simulink model "gm_mpu6050"  (R2017a)
settings: Solver=FixedStepDiscrete  StartTime=0.0  StopTime=0.004  RelTol=1e-3
PostLoadFcn:
  | ChipSelect = 1;  % choose I2C comms
  | AddressAlt = 0;  % use default address
  | 
  | if AddressAlt == 1
  | % b1101001 (pin AD0 is logic high).
  | SlvAddr = uint8(bin2dec('1101001'));  % ADDR ALT = 1
  | else
  | % b1101000 (pin AD0 is logic low)
  | SlvAddr = uint8(bin2dec('1101000'));  % ADDR ALT = 0
  | end
  | SlvAddr = uint8(hex2dec('68'));
  | 
  | 
  | % 0x3B 59 ACCEL_XOUT[15:8]
  | % 0x3C 60 ACCEL_XOUT[7:0]
  | % 0x3D 61 ACCEL_YOUT[15:8]
  | % 0x3E 62 ACCEL_YOUT[7:0]
  | % 0x3F 63 ACCEL_ZOUT[15:8]
  | % 0x40 64 ACCEL_ZOUT[7:0]
  | 
  | AccelXRegAddr = uint8(hex2dec('3B'));
  | AccelYRegAddr = uint8(hex2dec('3D'));
  | AccelZRegAddr = uint8(hex2dec('3F'));
  | 
  | % 0x43 67 GYRO_XOUT[15:8]
  | % 0x44 68 GYRO_XOUT[7:0]
  | % 0x45 69 GYRO_YOUT[15:8]
  | % 0x46 70 GYRO_YOUT[7:0]
  | % 0x47 71 GYRO_ZOUT[15:8]
  | % 0x48 72 GYRO_ZOUT[7:0]
  | 
  | GyroXRegAddr = uint8(hex2dec('43'));
  | GyroYRegAddr = uint8(hex2dec('45'));
  | GyroZRegAddr = uint8(hex2dec('47'));
  | 
  | deviceAddr = fi(SlvAddr,0,7,0);
  | 
  | powerRegAddr = uint8(hex2dec('6B'));
  | powerRegData = bin2dec('10000001');
settings Model: Creator=skuznick  LastModifiedBy=mini
settings DataIOCC: SaveOutput=off  SaveTime=off
settings OptimizationCC: BlockReduction=off  ConditionallyExecuteInputs=off  DefaultParameterBehavior=Inlined
settings DebuggingCC: AlgebraicLoopMsg=error  InheritedTsInSrcMsg=none  SingleTaskRateTransMsg=error
settings HardwareCC: ProdBitPerPointer=32  ProdBitPerSizeT=32  ProdBitPerPtrDiffT=32  ProdLargestAtomicFloat=None  ProdIntDivRoundTo=Undefined  ProdEndianess=Unspecified  ProdWordSize=32  ProdHWDeviceType=ASIC/FPGA->ASIC/FPGA  ProdEqTarget=off
settings GRTTargetCC: ExtMode=on

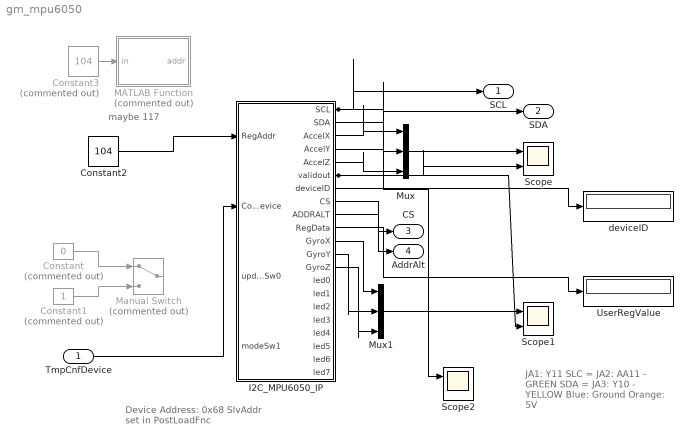
== system gm_mpu6050 ==
  note: Device Address: 0x68
      | SlvAddr set in PostLoadFnc
  note: JA1: Y11
      | SLC = JA2: AA11 - GREEN
      | SDA = JA3: Y10  - YELLOW
      | Blue: Ground
      | Orange: 5V
  note: maybe 117
  TmpCnfDevice : Inport  OutDataTypeStr=boolean
  Constant : Constant  Commented=on  Value=0  OutDataTypeStr=boolean  SampleTime=-1
  Constant1 : Constant  Commented=on  OutDataTypeStr=boolean  SampleTime=-1
  Constant2 : Constant  Value=104  OutDataTypeStr=uint8  SampleTime=-1
  Constant3 : Constant  Commented=on  Value=104  OutDataTypeStr=uint8  SampleTime=-1
  I2C_MPU6050_IP : Subsystem  TreatAsAtomicUnit=on  SystemSampleTime=1/400e3
  MATLAB Function : MATLAB Function  Commented=on  TreatAsAtomicUnit=on
  Manual Switch : ManualSwitch  Commented=on
  Mux : Mux  Inputs=3
  Mux1 : Mux  Inputs=3
  Scope : Scope  NumInputPorts=2
  Scope1 : Scope  NumInputPorts=2
  Scope2 : Scope  NumInputPorts=2
  UserRegValue : Display
  deviceID : Display
  SCL : Outport
  SDA : Outport  Port=2
  CS : Outport  Port=3
  AddrAlt : Outport  Port=4
  wires:
  Constant3/1 -> MATLAB Function/1(in)
  TmpCnfDevice/1 -> I2C_MPU6050_IP/2(ConfigDevice)
  I2C_MPU6050_IP/6(validout) -> Scope1/2, Scope/2
  I2C_MPU6050_IP/12(GyroY) -> Mux1/2
  I2C_MPU6050_IP/11(GyroX) -> Mux1/1
  I2C_MPU6050_IP/13(GyroZ) -> Mux1/3
  Mux1/1 -> Scope1/1
  Constant2/1 -> I2C_MPU6050_IP/1(RegAddr)
  Constant1/1 -> Manual Switch/2
  Constant/1 -> Manual Switch/1
  Mux/1 -> Scope/1
  I2C_MPU6050_IP/10(RegData) -> UserRegValue/1
  I2C_MPU6050_IP/7(deviceID) -> deviceID/1
  I2C_MPU6050_IP/5(AccelZ) -> Mux/3
  I2C_MPU6050_IP/3(AccelX) -> Mux/1
  I2C_MPU6050_IP/4(AccelY) -> Mux/2
  I2C_MPU6050_IP/9(ADDRALT) -> AddrAlt/1
  I2C_MPU6050_IP/8(CS) -> CS/1
  I2C_MPU6050_IP/1(SCL) -> SCL/1, Scope2/1
  I2C_MPU6050_IP/2(SDA) -> SDA/1

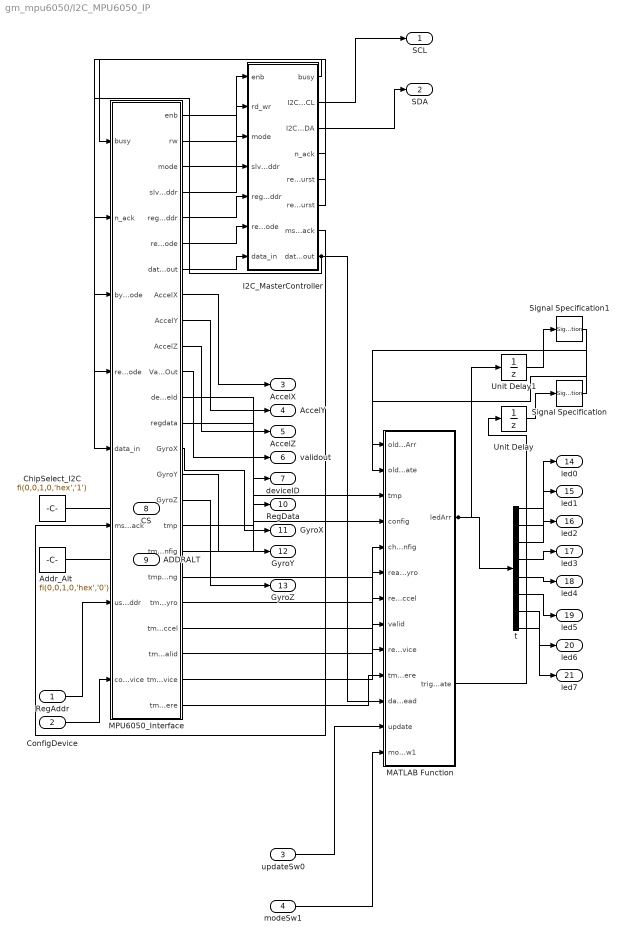
== system gm_mpu6050/I2C_MPU6050_IP ==
  RegAddr : Inport  OutDataTypeStr=uint8  SampleTime=2.5e-06
  ConfigDevice : Inport  Port=2  OutDataTypeStr=boolean  SampleTime=2.5e-06
  updateSw0 : Inport  Port=3  OutDataTypeStr=boolean  SampleTime=2.5e-06
  modeSw1 : Inport  Port=4  OutDataTypeStr=boolean  SampleTime=2.5e-06
  Addr_Alt : Constant  Value=fi(0,0,1,0,'hex','0')  OutDataTypeStr=boolean  SampleTime=-1
  ChipSelect_I2C : Constant  Value=fi(0,0,1,0,'hex','1')  OutDataTypeStr=boolean  SampleTime=-1
  I2C_MasterController : Subsystem
  MATLAB Function : Subsystem
  MPU6050_Interface : Subsystem
  Signal Specification : SignalSpecification  OutDataTypeStr=boolean  Dimensions=1
  Signal Specification1 : SignalSpecification  OutDataTypeStr=boolean  Dimensions=8
  Unit Delay : UnitDelay  SampleTime=2.5e-06
  Unit Delay1 : UnitDelay  SampleTime=2.5e-06
  t : Demux  Outputs=8
  SCL : Outport
  SDA : Outport  Port=2
  AccelX : Outport  Port=3
  AccelY : Outport  Port=4
  AccelZ : Outport  Port=5
  validout : Outport  Port=6
  deviceID : Outport  Port=7
  CS : Outport  Port=8
  ADDRALT : Outport  Port=9
  RegData : Outport  Port=10
  GyroX : Outport  Port=11
  GyroY : Outport  Port=12
  GyroZ : Outport  Port=13
  led0 : Outport  Port=14  OutDataTypeStr=boolean
  led1 : Outport  Port=15  OutDataTypeStr=boolean
  led2 : Outport  Port=16  OutDataTypeStr=boolean
  led3 : Outport  Port=17  OutDataTypeStr=boolean
  led4 : Outport  Port=18  OutDataTypeStr=boolean
  led5 : Outport  Port=19  OutDataTypeStr=boolean
  led6 : Outport  Port=20  OutDataTypeStr=boolean
  led7 : Outport  Port=21  OutDataTypeStr=boolean
  wires:
  RegAddr/1 -> MPU6050_Interface/7(userRegAddr)
  ConfigDevice/1 -> MPU6050_Interface/8(configDevice)
  updateSw0/1 -> MATLAB Function/12(update)
  modeSw1/1 -> MATLAB Function/13(modeSw1)
  Addr_Alt/1 -> ADDRALT/1
  ChipSelect_I2C/1 -> CS/1
  I2C_MasterController/1(busy) -> MPU6050_Interface/1(busy)
  I2C_MasterController/2(I2C_SCL) -> SCL/1
  I2C_MasterController/3(I2C_SDA) -> SDA/1
  I2C_MasterController/4(n_ack) -> MPU6050_Interface/2(n_ack)
  I2C_MasterController/5(reg_data_burst) -> MPU6050_Interface/3(byte_mode)
  I2C_MasterController/6(reg_addr_burst) -> MPU6050_Interface/4(reg_mode)
  I2C_MasterController/7(mstr_ack) -> MPU6050_Interface/6(mstr_ack)
  I2C_MasterController/8(data_out) -> MPU6050_Interface/5(data_in), MATLAB Function/11(dataRead)
  MATLAB Function/1(ledArr) -> t/1, Unit Delay1/1
  MATLAB Function/2(trigUpdate) -> Unit Delay/1
  MPU6050_Interface/1(enb) -> I2C_MasterController/1(enb)
  MPU6050_Interface/2(rw) -> I2C_MasterController/2(rd_wr)
  MPU6050_Interface/3(mode) -> I2C_MasterController/3(mode)
  MPU6050_Interface/4(slv_addr) -> I2C_MasterController/4(slv_addr)
  MPU6050_Interface/5(reg_addr) -> I2C_MasterController/5(reg_addr)
  MPU6050_Interface/6(reg_byte_mode) -> I2C_MasterController/6(reg_byte_mode)
  MPU6050_Interface/7(data_out) -> I2C_MasterController/7(data_in)
  MPU6050_Interface/8(AccelX) -> AccelX/1
  MPU6050_Interface/9(AccelY) -> AccelY/1
  MPU6050_Interface/10(AccelZ) -> AccelZ/1
  MPU6050_Interface/11(Valid_Out) -> validout/1
  MPU6050_Interface/12(deviceId) -> deviceID/1
  MPU6050_Interface/13(regdata) -> RegData/1
  MPU6050_Interface/14(GyroX) -> GyroX/1
  MPU6050_Interface/15(GyroY) -> GyroY/1
  MPU6050_Interface/16(GyroZ) -> GyroZ/1
  MPU6050_Interface/17(tmp) -> MATLAB Function/3(tmp)
  MPU6050_Interface/18(tmpConfig) -> MATLAB Function/4(config)
  MPU6050_Interface/19(tmpCheckCng) -> MATLAB Function/5(checkConfig)
  MPU6050_Interface/20(tmpReadGyro) -> MATLAB Function/6(readGyro)
  MPU6050_Interface/21(tmpReadAccel) -> MATLAB Function/7(readAccel)
  MPU6050_Interface/22(tmpValid) -> MATLAB Function/8(valid)
  MPU6050_Interface/23(tmpReadDevice) -> MATLAB Function/9(readDevice)
  MPU6050_Interface/24(tmpHere) -> MATLAB Function/10(tmpHere)
  Signal Specification/1 -> MATLAB Function/2(oldTrigUpdate)
  Signal Specification1/1 -> MATLAB Function/1(oldLedArr)
  Unit Delay/1 -> Signal Specification/1
  Unit Delay1/1 -> Signal Specification1/1
  t/1 -> led0/1
  t/2 -> led1/1
  t/3 -> led2/1
  t/4 -> led3/1
  t/5 -> led4/1
  t/6 -> led5/1
  t/7 -> led6/1
  t/8 -> led7/1

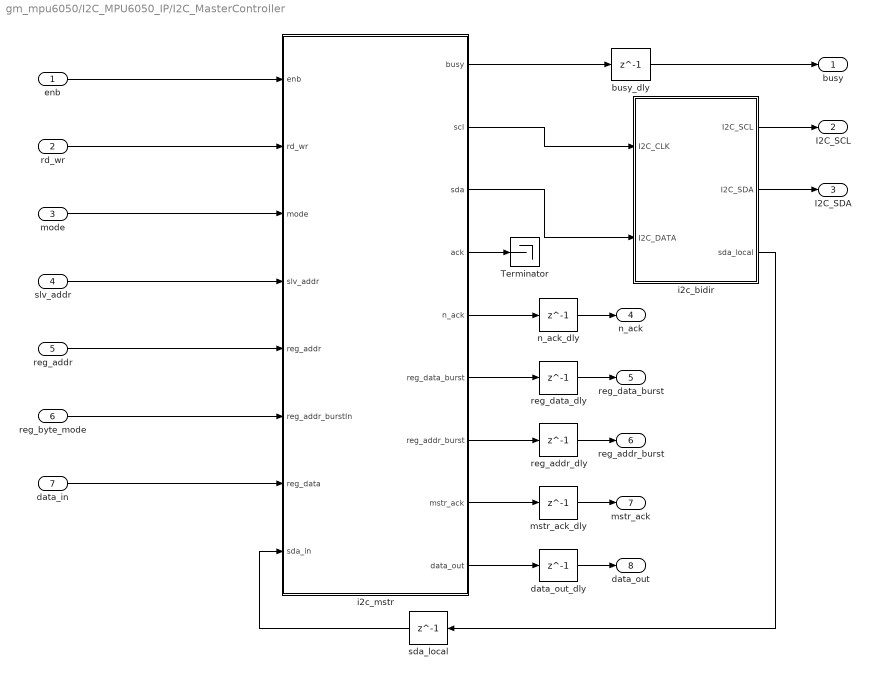
== system gm_mpu6050/I2C_MPU6050_IP/I2C_MasterController ==
  enb : Inport  SampleTime=2.5e-06
  rd_wr : Inport  Port=2  SampleTime=2.5e-06
  mode : Inport  Port=3  SampleTime=2.5e-06
  slv_addr : Inport  Port=4  SampleTime=2.5e-06
  reg_addr : Inport  Port=5  SampleTime=2.5e-06
  reg_byte_mode : Inport  Port=6  SampleTime=2.5e-06
  data_in : Inport  Port=7  SampleTime=2.5e-06
  Terminator : Terminator
  busy_dly : Delay  DelayLength=1
  data_out_dly : Delay  DelayLength=1
  i2c_bidir : Subsystem  TreatAsAtomicUnit=on
  i2c_mstr : Subsystem
  mstr_ack_dly : Delay  DelayLength=1
  n_ack_dly : Delay  DelayLength=1
  reg_addr_dly : Delay  DelayLength=1
  reg_data_dly : Delay  DelayLength=1
  sda_local : Delay  DelayLength=1
  busy : Outport
  I2C_SCL : Outport  Port=2
  I2C_SDA : Outport  Port=3
  n_ack : Outport  Port=4
  reg_data_burst : Outport  Port=5
  reg_addr_burst : Outport  Port=6
  mstr_ack : Outport  Port=7
  data_out : Outport  Port=8
  wires:
  enb/1 -> i2c_mstr/1(enb)
  rd_wr/1 -> i2c_mstr/2(rd_wr)
  mode/1 -> i2c_mstr/3(mode)
  slv_addr/1 -> i2c_mstr/4(slv_addr)
  reg_addr/1 -> i2c_mstr/5(reg_addr)
  reg_byte_mode/1 -> i2c_mstr/6(reg_addr_burstIn)
  data_in/1 -> i2c_mstr/7(reg_data)
  busy_dly/1 -> busy/1
  data_out_dly/1 -> data_out/1
  i2c_bidir/1(I2C_SCL) -> I2C_SCL/1
  i2c_bidir/2(I2C_SDA) -> I2C_SDA/1
  i2c_bidir/3(sda_local) -> sda_local/1
  i2c_mstr/1(busy) -> busy_dly/1
  i2c_mstr/2(scl) -> i2c_bidir/1(I2C_CLK)
  i2c_mstr/3(sda) -> i2c_bidir/2(I2C_DATA)
  i2c_mstr/4(ack) -> Terminator/1
  i2c_mstr/5(n_ack) -> n_ack_dly/1
  i2c_mstr/6(reg_data_burst) -> reg_data_dly/1
  i2c_mstr/7(reg_addr_burst) -> reg_addr_dly/1
  i2c_mstr/8(mstr_ack) -> mstr_ack_dly/1
  i2c_mstr/9(data_out) -> data_out_dly/1
  mstr_ack_dly/1 -> mstr_ack/1
  n_ack_dly/1 -> n_ack/1
  reg_addr_dly/1 -> reg_addr_burst/1
  reg_data_dly/1 -> reg_data_burst/1
  sda_local/1 -> i2c_mstr/8(sda_in)

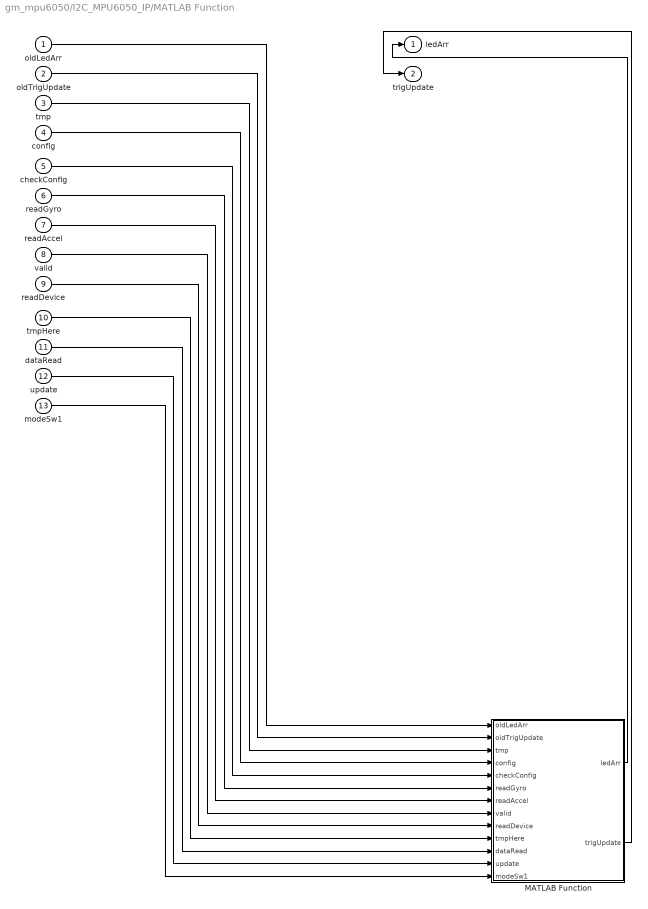
== system gm_mpu6050/I2C_MPU6050_IP/MATLAB Function ==
  oldLedArr : Inport  PortDimensions=[1, 8]  SampleTime=2.5e-06
  oldTrigUpdate : Inport  Port=2  SampleTime=2.5e-06
  tmp : Inport  Port=3  SampleTime=2.5e-06
  config : Inport  Port=4  SampleTime=2.5e-06
  checkConfig : Inport  Port=5  SampleTime=2.5e-06
  readGyro : Inport  Port=6  SampleTime=2.5e-06
  readAccel : Inport  Port=7  SampleTime=2.5e-06
  valid : Inport  Port=8  SampleTime=2.5e-06
  readDevice : Inport  Port=9  SampleTime=2.5e-06
  tmpHere : Inport  Port=10  SampleTime=2.5e-06
  dataRead : Inport  Port=11  SampleTime=2.5e-06
  update : Inport  Port=12  SampleTime=2.5e-06
  modeSw1 : Inport  Port=13  SampleTime=2.5e-06
  MATLAB Function : MATLAB Function  TreatAsAtomicUnit=on
  ledArr : Outport
  trigUpdate : Outport  Port=2
  wires:
  oldLedArr/1 -> MATLAB Function/1(oldLedArr)
  oldTrigUpdate/1 -> MATLAB Function/2(oldTrigUpdate)
  tmp/1 -> MATLAB Function/3(tmp)
  config/1 -> MATLAB Function/4(config)
  checkConfig/1 -> MATLAB Function/5(checkConfig)
  readGyro/1 -> MATLAB Function/6(readGyro)
  readAccel/1 -> MATLAB Function/7(readAccel)
  valid/1 -> MATLAB Function/8(valid)
  readDevice/1 -> MATLAB Function/9(readDevice)
  tmpHere/1 -> MATLAB Function/10(tmpHere)
  dataRead/1 -> MATLAB Function/11(dataRead)
  update/1 -> MATLAB Function/12(update)
  modeSw1/1 -> MATLAB Function/13(modeSw1)
  MATLAB Function/1(ledArr) -> ledArr/1
  MATLAB Function/2(trigUpdate) -> trigUpdate/1

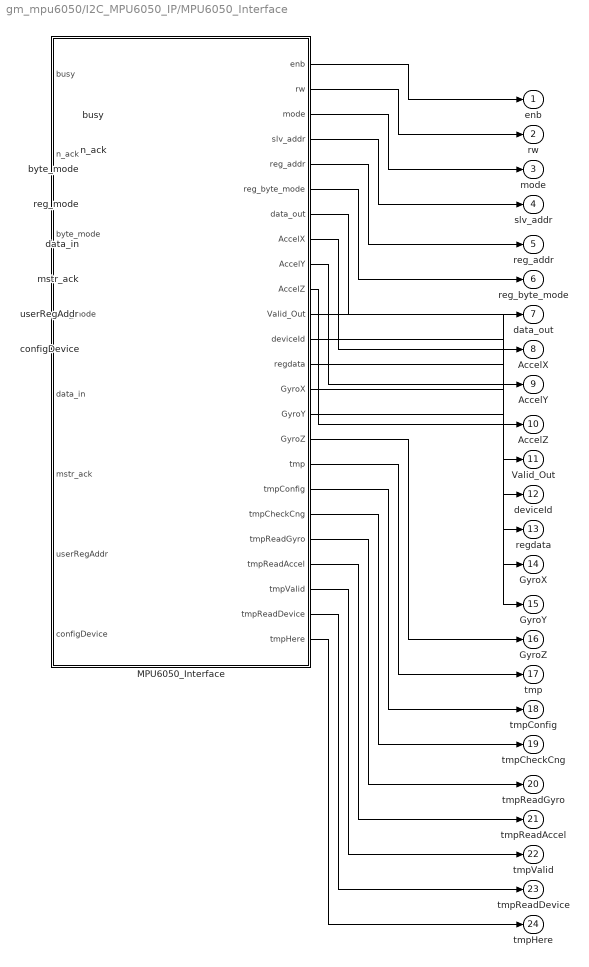
== system gm_mpu6050/I2C_MPU6050_IP/MPU6050_Interface ==
  busy : Inport  SampleTime=2.5e-06
  n_ack : Inport  Port=2  SampleTime=2.5e-06
  byte_mode : Inport  Port=3  SampleTime=2.5e-06
  reg_mode : Inport  Port=4  SampleTime=2.5e-06
  data_in : Inport  Port=5  SampleTime=2.5e-06
  mstr_ack : Inport  Port=6  SampleTime=2.5e-06
  userRegAddr : Inport  Port=7  SampleTime=2.5e-06
  configDevice : Inport  Port=8  SampleTime=2.5e-06
  MPU6050_Interface : Stateflow chart  TreatAsAtomicUnit=on
  enb : Outport
  rw : Outport  Port=2
  mode : Outport  Port=3
  slv_addr : Outport  Port=4
  reg_addr : Outport  Port=5
  reg_byte_mode : Outport  Port=6
  data_out : Outport  Port=7
  AccelX : Outport  Port=8
  AccelY : Outport  Port=9
  AccelZ : Outport  Port=10
  Valid_Out : Outport  Port=11
  deviceId : Outport  Port=12
  regdata : Outport  Port=13
  GyroX : Outport  Port=14
  GyroY : Outport  Port=15
  GyroZ : Outport  Port=16
  tmp : Outport  Port=17
  tmpConfig : Outport  Port=18
  tmpCheckCng : Outport  Port=19
  tmpReadGyro : Outport  Port=20
  tmpReadAccel : Outport  Port=21
  tmpValid : Outport  Port=22
  tmpReadDevice : Outport  Port=23
  tmpHere : Outport  Port=24
  wires:
  busy/1 -> MPU6050_Interface/1(busy)
  n_ack/1 -> MPU6050_Interface/2(n_ack)
  byte_mode/1 -> MPU6050_Interface/3(byte_mode)
  reg_mode/1 -> MPU6050_Interface/4(reg_mode)
  data_in/1 -> MPU6050_Interface/5(data_in)
  mstr_ack/1 -> MPU6050_Interface/6(mstr_ack)
  userRegAddr/1 -> MPU6050_Interface/7(userRegAddr)
  configDevice/1 -> MPU6050_Interface/8(configDevice)
  MPU6050_Interface/1(enb) -> enb/1
  MPU6050_Interface/2(rw) -> rw/1
  MPU6050_Interface/3(mode) -> mode/1
  MPU6050_Interface/4(slv_addr) -> slv_addr/1
  MPU6050_Interface/5(reg_addr) -> reg_addr/1
  MPU6050_Interface/6(reg_byte_mode) -> reg_byte_mode/1
  MPU6050_Interface/7(data_out) -> data_out/1
  MPU6050_Interface/8(AccelX) -> AccelX/1
  MPU6050_Interface/9(AccelY) -> AccelY/1
  MPU6050_Interface/10(AccelZ) -> AccelZ/1
  MPU6050_Interface/11(Valid_Out) -> Valid_Out/1
  MPU6050_Interface/12(deviceId) -> deviceId/1
  MPU6050_Interface/13(regdata) -> regdata/1
  MPU6050_Interface/14(GyroX) -> GyroX/1
  MPU6050_Interface/15(GyroY) -> GyroY/1
  MPU6050_Interface/16(GyroZ) -> GyroZ/1
  MPU6050_Interface/17(tmp) -> tmp/1
  MPU6050_Interface/18(tmpConfig) -> tmpConfig/1
  MPU6050_Interface/19(tmpCheckCng) -> tmpCheckCng/1
  MPU6050_Interface/20(tmpReadGyro) -> tmpReadGyro/1
  MPU6050_Interface/21(tmpReadAccel) -> tmpReadAccel/1
  MPU6050_Interface/22(tmpValid) -> tmpValid/1
  MPU6050_Interface/23(tmpReadDevice) -> tmpReadDevice/1
  MPU6050_Interface/24(tmpHere) -> tmpHere/1

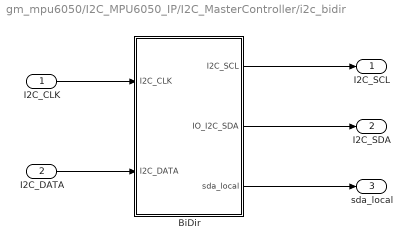
== system gm_mpu6050/I2C_MPU6050_IP/I2C_MasterController/i2c_bidir ==
  I2C_CLK : Inport
  I2C_DATA : Inport  Port=2
  BiDir : Subsystem  TreatAsAtomicUnit=on
  I2C_SCL : Outport
  I2C_SDA : Outport  Port=2
  sda_local : Outport  Port=3
  wires:
  BiDir/3(sda_local) -> sda_local/1
  BiDir/1("I2C_SCL ") -> I2C_SCL/1
  I2C_DATA/1 -> BiDir/2(I2C_DATA)
  I2C_CLK/1 -> BiDir/1(I2C_CLK)
  BiDir/2(IO_I2C_SDA) -> I2C_SDA/1

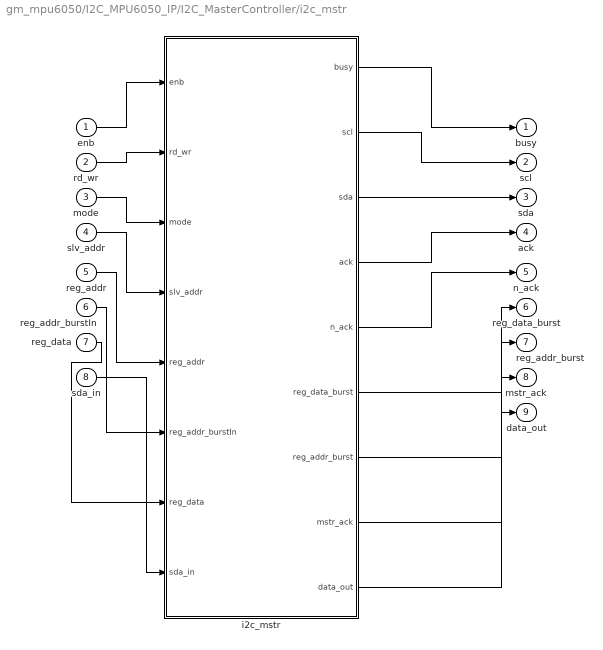
== system gm_mpu6050/I2C_MPU6050_IP/I2C_MasterController/i2c_mstr ==
  enb : Inport  SampleTime=2.5e-06
  rd_wr : Inport  Port=2  SampleTime=2.5e-06
  mode : Inport  Port=3  SampleTime=2.5e-06
  slv_addr : Inport  Port=4  SampleTime=2.5e-06
  reg_addr : Inport  Port=5  SampleTime=2.5e-06
  reg_addr_burstIn : Inport  Port=6  SampleTime=2.5e-06
  reg_data : Inport  Port=7  SampleTime=2.5e-06
  sda_in : Inport  Port=8  SampleTime=2.5e-06
  i2c_mstr : Stateflow chart  TreatAsAtomicUnit=on
  busy : Outport
  scl : Outport  Port=2
  sda : Outport  Port=3
  ack : Outport  Port=4
  n_ack : Outport  Port=5
  reg_data_burst : Outport  Port=6
  reg_addr_burst : Outport  Port=7
  mstr_ack : Outport  Port=8
  data_out : Outport  Port=9
  wires:
  enb/1 -> i2c_mstr/1(enb)
  rd_wr/1 -> i2c_mstr/2(rd_wr)
  mode/1 -> i2c_mstr/3(mode)
  slv_addr/1 -> i2c_mstr/4(slv_addr)
  reg_addr/1 -> i2c_mstr/5(reg_addr)
  reg_addr_burstIn/1 -> i2c_mstr/6(reg_addr_burstIn)
  reg_data/1 -> i2c_mstr/7(reg_data)
  sda_in/1 -> i2c_mstr/8(sda_in)
  i2c_mstr/1(busy) -> busy/1
  i2c_mstr/2(scl) -> scl/1
  i2c_mstr/3(sda) -> sda/1
  i2c_mstr/4(ack) -> ack/1
  i2c_mstr/5(n_ack) -> n_ack/1
  i2c_mstr/6(reg_data_burst) -> reg_data_burst/1
  i2c_mstr/7(reg_addr_burst) -> reg_addr_burst/1
  i2c_mstr/8(mstr_ack) -> mstr_ack/1
  i2c_mstr/9(data_out) -> data_out/1

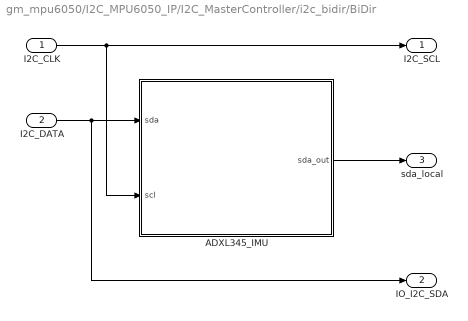
== system gm_mpu6050/I2C_MPU6050_IP/I2C_MasterController/i2c_bidir/BiDir ==
  I2C_CLK : Inport  OutDataTypeStr=boolean
  I2C_DATA : Inport  Port=2  OutDataTypeStr=boolean
  ADXL345_IMU : Stateflow chart  TreatAsAtomicUnit=on
  "I2C_SCL " : Outport  OutDataTypeStr=boolean
  IO_I2C_SDA : Outport  Port=2  OutDataTypeStr=boolean
  sda_local : Outport  Port=3  OutDataTypeStr=boolean
  wires:
  I2C_DATA/1 -> ADXL345_IMU/1(sda), IO_I2C_SDA/1
  I2C_CLK/1 -> ADXL345_IMU/2(scl), "I2C_SCL "/1
  ADXL345_IMU/1(sda_out) -> sda_local/1

== stateflow chart gm_mpu6050/I2C_MPU6050_IP/MPU6050_Interface/MPU6050_Interface ==
  settings: executeAtInitialization=1
  state init
    %initstate
    Valid_Out = 0;
    selfInit = 1;
    slv_addr = SlvAddr;
    %TODO delete all
    tmp = 0;
    tmpConfig = 0;
    tmpReadGyro = 0;
    tmpReadAccel = 0;
    tmpValid = 0;
    tmpReadDevice = 0;
    tmpHere = 0;
  note: I2C Configuration for MPU6050
  note: 0x3B 59 ACCEL_XOUT[15:8]
      | 0x3C 60 ACCEL_XOUT[7:0]
      | 0x3D 61 ACCEL_YOUT[15:8]
      | 0x3E 62 ACCEL_YOUT[7:0]
      | 0x3F 63 ACCEL_ZOUT[15:8]
      | 0x40 64 ACCEL_ZOUT[7:0]
      |
      | 0x43 67 GYRO_XOUT[15:8]
      | 0x44 68 GYRO_XOUT[7:0]
      | 0x45 69 GYRO_YOUT[15:8]
      | 0x46 70 GYRO_YOUT[7:0]
      | 0x47 71 GYRO_ZOUT[15:8]
      | 0x48 72 GYRO_ZOUT[7:0]
      |
      | 0x6B 107 PWR_MGMT_1
      | 0x6C 108 PWR_MGMT_2
  state idle
    %idlestate
    enb 	= 0;
    rw 		= 0;
    mode 	= 0;
    cnt      = 0;
    reg_byte_mode = 0;
  state ReadDeviceData [group]
    note: DEVID is an example of
        | doing a 1-byte READ
    note: 0x75 117 - WHO_AM_I[6:1]
    state getDEVID
      entry:
      enb = 1;
      rw = 1;
      mode = 0;
      reg_addr =   uint8(117);
      tmpReadDevice = 1;
    state waitforNotBusy1
      enb=0;
    state readDEVID
      deviceId = uint8(data_in);
      tmpHere = 1;
    state waitforNotBusy6
      enb=0;
    state getRegData
      entry:
      enb = 1;
      rw = 1;
      mode = 0;
      reg_addr = userRegAddr;
    state waitforNotBusy5
      enb=0;
    state readUserRegData
      regdata = uint8(data_in);
    getDEVID -> waitforNotBusy1 : [busy==1]
    waitforNotBusy1 -> readDEVID [order 1] : [mstr_ack==1]
    waitforNotBusy1 -> waitforNotBusy6 [order 2] : [n_ack==1]
    readDEVID -> getRegData : [busy==0]
    waitforNotBusy6 -> (junction 2281) : [busy==0 || busy == 1]
    getRegData -> waitforNotBusy5 : [busy==1]
    waitforNotBusy5 -> readUserRegData [order 1] : [mstr_ack==1]
    waitforNotBusy5 -> (junction 2281) [order 2] : [n_ack==1]
  state Configuration [group]
    state setPwrMode
      enb = 1;
      rw = 0;
      mode = 0;
      reg_addr = powerRegAddr;
      data_out = powerRegData;
      tmpConfig = 1;
    state waitforNotBusy2
      enb=0;
    state setDataFormat [commented out]
      enb = 1;
      rw = 0;
      mode = 0;
      reg_addr = uint8(49); % 0x31
      data_out = uint8(0); % or 0x08
    state waitforNotBusy3 [commented out]
      enb=0;
    state setFIFOCfg [commented out]
      enb = 1;
      rw = 0;
      mode = 0;
      reg_addr = uint8(56); % 0x38
      data_out = uint8(8); % 0x08
    state waitforNotBusy4 [commented out]
      enb=0;
    state cfgDone
      selfInit = 0;
      tmp = 1;
    setPwrMode -> Configuration.waitforNotBusy2 : [busy==1]
    Configuration.waitforNotBusy2 -> (junction 2329) [order 2] : [busy==0]
    Configuration.waitforNotBusy2 -> (junction 2279) [order 1] : [n_ack==1]
    waitforNotBusy3 -> (junction 2279) [commented out] : [n_ack==1]
    waitforNotBusy4 -> (junction 2279) [commented out] : [n_ack==1]
    setDataFormat -> waitforNotBusy3 [commented out] : [busy==1]
    waitforNotBusy3 -> setFIFOCfg [commented out] : [busy==0]
    (junction 2329) -> cfgDone
    setFIFOCfg -> waitforNotBusy4 [commented out] : [busy==1]
  state check_cfg
    en: enb = 0;
    cnt = 0;
    du: cnt = cnt + 1;
    tmpCheckCng = 1
  state ReadAccelData [group]
    state read_accelX_registers0
      entry:
      enb = 1;
      rw = 1;
      mode = 1;
      reg_addr =  AccelXRegAddr;
      Valid_Out = 0;
      tmpReadAccel = 1;
    state waitforNotBusy2
      enb=0;
    state accelX_LSB
      tempVal = data_in;
    state toggle
    state accelX_MSB
      AccelX =  convert_int16(tempVal, data_in);
    state toggle3
    state accelY_LSB
      tempVal = data_in;
    state toggle1
    state accelY_MSB
      AccelY = convert_int16(tempVal,data_in);
    state toggle4
    state accelZ_LSB
      tempVal = data_in;
    state toggle2
      mode = 0;
    state accelZ_MSB
      AccelZ =  convert_int16(tempVal, data_in);
    read_accelX_registers0 -> ReadAccelData.waitforNotBusy2 : [busy==1]
    ReadAccelData.waitforNotBusy2 -> accelX_LSB [order 1] : [mstr_ack==1]
    accelX_LSB -> ReadAccelData.toggle : [mstr_ack==0]
    ReadAccelData.toggle -> accelX_MSB : [mstr_ack==1]
    accelX_MSB -> ReadAccelData.toggle3 [order 2] : [mstr_ack==0]
    accelX_MSB -> (junction 2286) [order 1] : [n_ack==1]
    ReadAccelData.toggle3 -> accelY_LSB : [mstr_ack==1]
    accelY_LSB -> ReadAccelData.toggle1 : [mstr_ack==0]
    ReadAccelData.toggle1 -> accelY_MSB : [mstr_ack==1]
    accelY_MSB -> (junction 2286) [order 1] : [n_ack==1]
    accelZ_MSB -> (junction 2286) [order 1] : [n_ack==1]
    accelY_MSB -> ReadAccelData.toggle4 [order 2] : [mstr_ack==0]
    ReadAccelData.toggle4 -> accelZ_LSB : [mstr_ack==1]
    accelZ_LSB -> ReadAccelData.toggle2 : [mstr_ack==0]
    ReadAccelData.toggle2 -> accelZ_MSB : [mstr_ack==1]
  state Valid
    en: enb = 0;
    cnt = 0;
    Valid_Out = 1;
    du: cnt = cnt + 1;
    tmpValid = 1;
  state ReadGyroData [group]
    state read_gyroX_registers0
      entry:
      enb = 1;
      rw = 1;
      mode = 1;
      reg_addr =  GyroXRegAddr;
      Valid_Out = 0;
      tmpReadGyro = 1;
    state waitforNotBusy2
      enb=0;
    state gyroX_LSB
      tempVal = data_in;
    state toggle
    state gyroX_MSB
      GyroX =  convert_int16(tempVal, data_in);
    state toggle3
    state gyroY_LSB
      tempVal = data_in;
    state toggle1
    state gyroY_MSB
      GyroY = convert_int16(tempVal, data_in);
    state toggle4
    state gyroZ_LSB
      tempVal = data_in;
    state toggle2
      mode = 0;
    state gyroZ_MSB
      GyroZ =  convert_int16(tempVal, data_in);
    read_gyroX_registers0 -> ReadGyroData.waitforNotBusy2 : [busy==1]
    ReadGyroData.waitforNotBusy2 -> gyroX_LSB : [mstr_ack==1]
    gyroX_LSB -> ReadGyroData.toggle : [mstr_ack==0]
    ReadGyroData.toggle -> gyroX_MSB : [mstr_ack==1]
    gyroX_MSB -> ReadGyroData.toggle3 [order 2] : [mstr_ack==0]
    gyroX_MSB -> (junction 2301) [order 1] : [n_ack==1]
    ReadGyroData.toggle3 -> gyroY_LSB : [mstr_ack==1]
    gyroY_LSB -> ReadGyroData.toggle1 : [mstr_ack==0]
    ReadGyroData.toggle1 -> gyroY_MSB : [mstr_ack==1]
    gyroY_MSB -> (junction 2301) [order 1] : [n_ack==1]
    gyroZ_MSB -> (junction 2301) [order 1] : [n_ack==1]
    gyroY_MSB -> ReadGyroData.toggle4 [order 2] : [mstr_ack==0]
    ReadGyroData.toggle4 -> gyroZ_LSB : [mstr_ack==1]
    gyroZ_LSB -> ReadGyroData.toggle2 : [mstr_ack==0]
    ReadGyroData.toggle2 -> gyroZ_MSB : [mstr_ack==1]
  (default) -> init
  init -> idle
  check_cfg -> idle : [cnt >=5]
  idle -> setPwrMode [order 1] : [busy==0 & (configDevice==1 | selfInit == 1)]
  idle -> getDEVID [order 2] : [busy==0]
  readUserRegData -> read_accelX_registers0 : [busy==0]
  (junction 2281) -> check_cfg
  (junction 2286) -> check_cfg
  (junction 2279) -> check_cfg
  ReadAccelData.waitforNotBusy2 -> check_cfg [order 2] : [n_ack==1]
  Valid -> check_cfg : [cnt >= 5]
  cfgDone -> read_accelX_registers0
  accelZ_MSB -> read_gyroX_registers0 [order 2] : [busy==0]
  gyroZ_MSB -> Valid [order 2]
  data: msb function_input uint8; lsb function_input uint8; val function_output int16; enb output boolean size=1; rw output boolean size=1; mode output boolean size=1; slv_addr output uint8; reg_addr output uint8; reg_byte_mode output boolean size=1; data_out output uint8; busy input; n_ack input; byte_mode input boolean size=1; reg_mode input boolean size=1; cnt local uint32; data_in input uint8 size=1; mstr_ack input; AccelX output int16; AccelY output int16; AccelZ output int16; SlvAddr parameter uint8; AccelXRegAddr parameter uint8; AccelYRegAddr parameter uint8; AccelZRegAddr parameter uint8; Valid_Out output boolean; tempVal local uint8; deviceId output uint8; powerRegData parameter uint8; regdata output uint8; userRegAddr input uint8; powerRegAddr parameter uint8; configDevice input boolean; selfInit local boolean; GyroXRegAddr parameter uint8; GyroX output int16; GyroY output int16; GyroZ output int16; tmp output boolean; tmpConfig output boolean; tmpCheckCng output boolean; tmpReadGyro output boolean; tmpReadAccel output boolean; tmpValid output boolean; tmpReadDevice output boolean; tmpHere output boolean
  function val = convert_int16(msb, lsb):
    | function val = convert_int16(msb, lsb)
    | 
    | val = int16(bitor(bitshift(int16(msb),8), int16(lsb)));

== stateflow chart gm_mpu6050/I2C_MPU6050_IP/I2C_MasterController/i2c_mstr/i2c_mstr ==
  settings: executeAtInitialization=1
  state idle
    entry:
    scl(:) = 1;
    sda(:) = 1;
    busy(:)  = 0;
    reg_data_burst(:) = 0;
    temp_data = uint8(0);
  note: I2C Master Controller
  state stop_ext
    entry:
    scl (:) = 1;
    sda(:) = 1;
    ack(:) = 0;
  state ready
    entry:
    scl(:) = 1;
    sda(:) = 1;
    data_out(:) = 0;
  state stop
    entry:
    sda(:) = 0;
  state start_n
    entry:
    scl(:) = 1;
    sda(:) = 0;
    bit_cnt(:) = 7;
    busy(:) = 1;
    reg_byte_cnt =1;
    data_out(:) = 0;
  state mastr_ack_data_cnf1
    entry:
    scl(:) = 1;
    sda(:) = 1;
    mstr_ack (:) = 1;
  state mastr_ack_data_cnf
    entry:
    scl(:) = 1;
    sda(:) = 0;
    mstr_ack (:) = 1;
  state scl_ext_p
    entry:
    scl(:) = 1;
    sda(:) = 0;
    ack(:) = 0;
  state start_p
    entry:
    sda(:) = 0;
  state scl_ext_n
    entry:
    scl(:) = 0;
    sda(:) = 0;
    ack(:) = 0;
    mstr_ack(:) = 0;
  state mastr_ack_data
    entry:
    scl(:) = 0;
    if mode == 1
    sda(:) = 0; %ACK
    else
    sda(:) = 1; %NACK
    end
    mstr_ack(:) = 1;
    ack(:) = 0;
    data_out(:) = temp_data;
    temp_data(:) = 0;
  state cmd_slave_addr_n
    entry:
    scl(:) = 0;
    sda(:) = bitget(slv_addr(:),bit_cnt);
  state Increment_Byte_count1
    entry:
    scl(:) = 0;
    bit_cnt = 8;
    mstr_ack(:) =0;
    reg_data_burst(:) = 1;
    sda(:) = 1;
  state cmd_slave_addr_p
    entry:
    scl(:) = 1;
    bit_cnt = bit_cnt-1;
  state write_n
    entry:
    scl(:) = 0;
    sda(:) = 0;
  state ack_end1
    entry: scl(:)=1;
    sda(:)=1;
    ack(:)=1;
  state cmd_reg_read_data_p
    entry:
    scl(:) = 1;
    if sda_in == 1;
    temp_data = bitset(temp_data,bit_cnt);
    end
    bit_cnt = bit_cnt-1;
  state ack_end
    entry: scl(:)=1;
    sda(:)=1;
    ack(:)=1;
  state write_p
    entry:
    scl(:) = 1;
    sda(:) = 0;
  state ack_recv_wr3
    entry: scl(:)=1;
    sda(:)=1;
    ack(:)=1;
  state ack_data
    entry:
    scl(:) = 0;
    sda(:) = 1;
    ack(:) = 1;
  state ack_slv
    entry:
    scl(:) = 0;
    ack(:) = 1;
    sda(:) = 1;
  state cmd_reg_read_data_n
    entry:
    scl(:) = 0;
    %mstr_ack(:) = 0
    ack(:) = 1;
  state ack_recv_wr
    entry: scl(:)=1;
    sda(:)=1;
    ack(:)=1;
    bit_cnt = 8;
  state cmd_reg_data_p
    entry:
    scl(:) = 1;
    bit_cnt = bit_cnt-1;
  state ack_addr_m_cnf
    entry:
    scl(:) = 0;
    if rd_wr == 1
    sda(:) = 1;
    else
    sda(:) = 0;
    end
    bit_cnt = 8;
    ack(:) = 0;
  state ack_wr_p
    entry: scl(:)=0;
    ack(:)=0;
    sda(:)=0;
    bit_cnt = 8;
  state error_ack
    entry:
    scl(:) = 0;
    sda(:) = 1;
    n_ack(:) = 1;
  state cmd_reg_data_n
    entry:
    scl(:) = 0;
    ack(:) = 0;
    reg_data_burst(:) = 0;
    sda(:) = bitget(reg_data,bit_cnt);
  state delay
    entry:
    scl(:) = 0;
    sda(:) = 1;
  state cmd_reg_addr_n
    entry:
    scl(:) = 0;
    ack(:) = 0;
    sda(:) = bitget(reg_addr,bit_cnt);
    reg_addr_burst(:)=0;
  state repeat_strt_n
    entry:
    scl(:) = 1;
    sda(:) = 0;
    bit_cnt(:) = 7;
    busy(:) = 1;
    reg_byte_cnt =1;
  state ready_repeated
    entry:
    scl(:) = 1;
    sda(:) = 1;
  state cmd_reg_addr_p
    entry:
    scl(:)= 1;
    bit_cnt = bit_cnt-1;
  state repeat_strt_p
    entry:
    sda(:) = 0;
  state ready_repeated_dummy
    entry:
    scl(:) = 1;
    sda(:) = 1;
  state ack_addr_m
    entry:
    scl(:) = 0;
    ack (:) = 1;
    sda(:) = 1;
  state ack_recv_wr1
    entry: scl(:)=1;
    sda(:)=1;
    ack(:)=1;
  state ack_recv_wr2
    entry: scl(:)=1;
    sda(:)=1;
    ack(:)=1;
  state cmd_slave_addr_n1
    entry:
    scl(:) = 0;
    sda(:) = bitget(slv_addr(:),bit_cnt);
  state cmd_slave_addr_p1
    entry:
    scl(:) = 1;
    bit_cnt = bit_cnt-1;
  state ack_addrm1
    entry:
    scl(:) = 1;
    ack(:) = 0;
    bit_cnt = 8;
    reg_addr_burst(:)=1;
  state read_n
    entry:
    scl(:) = 0;
    sda(:) = 1;
  state ack_wr_p2
    entry: scl(:)=0;
    ack(:)=1;
    sda(:)=1;
  state read_p
    entry:
    scl(:) = 1;
    sda(:) = 1;
    bit_cnt = 8;
  state ack_slv1
    entry:
    scl(:) = 0;
    ack(:) = 1;
    sda(:) = 1;
  state ack_slv_cnf1
    entry:
    scl(:)= 1;
    ack(:) = 1;
    bit_cnt = 8;
  (default) -> idle
  stop_ext -> idle
  idle -> ready : [enb==1]
  stop -> stop_ext
  ready -> start_n
  scl_ext_p -> stop
  mastr_ack_data_cnf1 -> scl_ext_n
  start_n -> start_p
  mastr_ack_data_cnf -> Increment_Byte_count1
  mastr_ack_data -> mastr_ack_data_cnf [order 1] : [mode==1]
  mastr_ack_data -> mastr_ack_data_cnf1 [order 2]
  scl_ext_n -> scl_ext_p
  start_p -> cmd_slave_addr_n
  cmd_slave_addr_p -> cmd_slave_addr_n [order 1] : [bit_cnt > 0]
  error_ack -> scl_ext_n
  (junction 2294) -> scl_ext_n [order 2]
  cmd_slave_addr_n -> cmd_slave_addr_p
  cmd_slave_addr_p -> write_n [order 2]
  Increment_Byte_count1 -> cmd_reg_read_data_n
  ack_end -> (junction 2294) [order 1] : [sda_in == 0]
  (junction 2294) -> cmd_reg_data_n [order 1] : [mode == 1]{bit_cnt=8;reg_data_burst(:)=1;ack(:)=0;}
  cmd_reg_read_data_p -> mastr_ack_data [order 2]
  write_n -> write_p
  ack_data -> ack_end1
  ack_end1 -> ack_end
  cmd_reg_read_data_p -> cmd_reg_read_data_n [order 1] : [bit_cnt > 0]
  ack_slv -> ack_recv_wr3
  write_p -> ack_slv
  ack_end -> error_ack [order 2]
  cmd_reg_read_data_n -> cmd_reg_read_data_p
  ack_recv_wr3 -> ack_recv_wr
  cmd_reg_data_p -> ack_data [order 2]
  ack_wr_p2 -> cmd_reg_read_data_n
  ack_recv_wr -> error_ack [order 2]
  cmd_reg_data_p -> cmd_reg_data_n [order 1] : [bit_cnt > 0]
  ack_recv_wr -> ack_wr_p [order 1] : [sda_in == 0]
  cmd_reg_data_n -> cmd_reg_data_p
  ack_addr_m_cnf -> cmd_reg_data_n [order 1] : [rd_wr==0]
  ack_recv_wr2 -> ack_addr_m_cnf [order 1] : [sda_in == 0]
  ack_recv_wr2 -> error_ack [order 2]
  ack_slv_cnf1 -> error_ack [order 2]
  ack_wr_p -> cmd_reg_addr_n
  ack_addr_m_cnf -> delay [order 2] : [rd_wr==1]
  delay -> ready_repeated
  ack_addrm1 -> cmd_reg_addr_n
  cmd_reg_addr_p -> cmd_reg_addr_n [order 1] : [bit_cnt > 0]
  ready_repeated_dummy -> repeat_strt_n
  cmd_reg_addr_n -> cmd_reg_addr_p
  repeat_strt_n -> repeat_strt_p
  ready_repeated -> ready_repeated_dummy
  cmd_reg_addr_p -> ack_addr_m [order 2]
  repeat_strt_p -> cmd_slave_addr_n1
  ack_recv_wr1 -> ack_recv_wr2
  ack_addr_m -> ack_recv_wr1 [order 2]
  ack_addr_m -> ack_addrm1 [order 1] : [reg_addr_burstIn ==1]
  cmd_slave_addr_p1 -> cmd_slave_addr_n1 [order 1] : [bit_cnt > 0]
  cmd_slave_addr_n1 -> cmd_slave_addr_p1
  cmd_slave_addr_p1 -> read_n [order 2]
  read_n -> read_p
  ack_slv_cnf1 -> ack_wr_p2 [order 1] : [sda_in == 0]
  read_p -> ack_slv1
  ack_slv1 -> ack_slv_cnf1
  data: enb input boolean size=1; rd_wr input boolean size=1; mode input boolean size=1; busy output boolean size=1; bit_cnt local uint8; scl output boolean size=1; sda output boolean size=1; slv_addr input uint8; reg_addr input uint8; reg_addr_burstIn input boolean size=1; reg_data input uint8; sda_in input boolean size=1; ack output boolean size=1; n_ack output boolean size=1; reg_byte_cnt local uint8; reg_data_burst output boolean size=1; reg_addr_burst output boolean size=1; mstr_ack output boolean size=1; data_out output fixdt(0,8,0) size=1; temp_data local uint8

== matlab function gm_mpu6050/I2C_MPU6050_IP/MATLAB Function/MATLAB Function ==
  data: ledArr output; oldLedArr input; oldTrigUpdate input; tmp input; config input; checkConfig input; readGyro input; readAccel input; valid input; readDevice input; tmpHere input; dataRead input; trigUpdate output; update input; modeSw1 input
function [ledArr, trigUpdate] = fcn(oldLedArr, oldTrigUpdate, tmp, config, checkConfig, readGyro, readAccel, valid, readDevice, tmpHere, dataRead, update, modeSw1)    
    if( update == true && oldTrigUpdate == false ) %sw0
        ledArr = [false, false, false, false, false, false, false, false];
        if( modeSw1 == true ) %sw1 = 0
            ledArr(1) = tmp; % led0
            ledArr(2) = config;
            ledArr(3) = checkConfig;
            ledArr(4) = readGyro;
            ledArr(5) = readAccel;
            ledArr(6) = valid;
            ledArr(7) = readDevice;
            ledArr(8) = tmpHere; % led7
        else % mode 1 sw1 = 1
            ledArr(1) = logical(bitget(dataRead,1)); % led0
            ledArr(2) = logical(bitget(dataRead,2));
            ledArr(3) = logical(bitget(dataRead,3));
            ledArr(4) = logical(bitget(dataRead,4));
            ledArr(5) = logical(bitget(dataRead,5));
            ledArr(6) = logical(bitget(dataRead,6));
            ledArr(7) = logical(bitget(dataRead,7));
            ledArr(8) = logical(bitget(dataRead,8)); % led7
        end
        trigUpdate = true;
    else
        ledArr = oldLedArr;
        trigUpdate = false;
    end

== stateflow chart gm_mpu6050/I2C_MPU6050_IP/I2C_MasterController/i2c_bidir/BiDir/ADXL345_IMU ==
  state init
    entry:
    rd_cnt = 0;
    reg_idx = 0;
  state idle
    entry:
    sda_out = false;
    addr = fi(0,0,7,0);
    data = fi(0,0,8,0);
  state regdata = sendregdata(reg) [function]
    (default) -> (junction 86)
    (junction 86) -> (junction 89) [order 1] : [reg ==AccelXRegAddr]
    (junction 86) -> (junction 88) [order 2]
    (junction 89) -> (junction 90) : {regdata = hex2dec('D2');}
    (junction 90) -> (junction 99)
    (junction 99) -> (junction 112)
    (junction 88) -> (junction 97) [order 1] : [reg==AccelYRegAddr]
    (junction 97) -> (junction 111) : {regdata = hex2dec('E1');}
    (junction 88) -> (junction 91) [order 2]
    (junction 111) -> (junction 112)
    (junction 112) -> (junction 103)
    (junction 91) -> (junction 106) [order 1] : [reg==AccelZRegAddr]
    (junction 106) -> (junction 109) : {regdata=hex2dec('2E');}
    (junction 91) -> (junction 127) [order 2]
    (junction 109) -> (junction 103)
    (junction 103) -> (junction 143)
    (junction 127) -> (junction 126) [order 1] : [reg ==AccelXRegAddr+1]
    (junction 127) -> (junction 128) [order 2]
    (junction 126) -> (junction 131) : {regdata = hex2dec('04');}
    (junction 131) -> (junction 143)
    (junction 143) -> (junction 130)
    (junction 128) -> (junction 142) [order 1] : [reg==AccelYRegAddr+1]
    (junction 142) -> (junction 154) : {regdata = hex2dec('FF');}
    (junction 128) -> (junction 140) [order 2]
    (junction 154) -> (junction 130)
    (junction 130) -> (junction 149)
    (junction 140) -> (junction 141) [order 1] : [reg==AccelZRegAddr+1]
    (junction 141) -> (junction 153) : {regdata=hex2dec('16');}
    (junction 140) -> (junction 196) [order 2]
    (junction 153) -> (junction 149)
    (junction 149) -> (junction 197)
    (junction 196) -> (junction 194) [order 1] : [reg==powerRegAddr]
    (junction 194) -> (junction 192) : {regdata=hex2dec('FE');}
    (junction 196) -> (junction 152) [order 2] : {regdata=bin2dec('11100101');}
        | % Return the Device ID
    (junction 192) -> (junction 197)
    (junction 197) -> (junction 152)
  state start
    en:
    bit_idx(:) = 7;
  state startgetaddr
  state NACK
    entry: sda_out(:) = 1;
  state getaddr
    entry:
    if sda == 1
    addr = bitset(addr,bit_idx);
    end
    bit_idx = bit_idx - 1;
  note: RegX (0x32/0x33) = 1234 (0x04d2)
      | RegY (0x34/0x35) = 4321 (0x10e1)
      | RegZ (0x36/0x37) = 5678 (0x162e)
  state endgetaddr
    entry: rw = sda;
  state sendack
    entry:
    sda_out(:) = 0;
    bit_idx = 8;
  state senddatastart
    entry: data(:) = sendregdata(reg_idx+rd_cnt);
    bit_idx = 8;
  state waitForStop
  state getdatastart
  state sendbyte
    entry:
    sda_out(:) = bitget(data,bit_idx);
  state getdata
    entry:
    if sda == 1
    data = bitset(data,bit_idx);
    end
    bit_idx = bit_idx - 1;
  state sendbit
    entry:  bit_idx = bit_idx - 1;
  state waitforPos
  state endgetdata
    entry:
    reg_idx = uint8(data)
    sda_out(:) = 0;
  state lookRestart
    entry:
  state waitstop1
  state waitEndOfAck
  state getcfgregstart
  state sendAck
    entry: sda_out(:)=0;
    data
  state getcfgdata
    entry:
    if sda == 1
    data = bitset(data,bit_idx);
    end
    bit_idx = bit_idx - 1;
  (default) -> init
  init -> idle
  waitForStop -> idle : [scl==1 & sda==1]
  NACK -> idle
  idle -> start : [scl==1 & sda == 0]
  (junction 229) -> start [order 1] : [scl==1]
  start -> startgetaddr : [scl == 1]
  getaddr -> startgetaddr [order 1] : [bit_idx > 0]
  startgetaddr -> getaddr : [scl==1]
  endgetaddr -> NACK [order 1] : [addr ~= deviceAddr]
  getaddr -> endgetaddr [order 2] : [scl==1]
  endgetaddr -> sendack [order 2] : [scl==1]
  sendack -> senddatastart [order 1] : [scl==0 & rw==1]
  sendack -> getdatastart [order 2] : [scl==1 & rw==0] {rd_cnt=0;}
  waitstop1 -> senddatastart [order 2] : [scl==1&sda==0] {rd_cnt = rd_cnt + 1;}
  senddatastart -> sendbyte
  waitstop1 -> waitForStop [order 1] : [scl==1&sda==1]
  waitEndOfAck -> waitForStop : [scl==1&sda==0]
  getdata -> getdatastart [order 1] : [bit_idx > 0]
  getdatastart -> getdata : [scl == 1]
  sendbit -> sendbyte [order 1] : [bit_idx > 0]
  sendbyte -> sendbit : [scl==1]
  (junction 229) -> getcfgdata [order 2] : [scl==0] {bit_idx(:)=8;data(:)=0;}
  lookRestart -> (junction 229) : [sda==0]
  getdata -> endgetdata [order 2] : [scl==1]
  sendbit -> waitstop1 [order 2] : [scl==0]
  endgetdata -> waitforPos : [scl==1]
  waitforPos -> lookRestart [order 2] : [scl==1&sda==1]
  waitforPos -> getcfgdata [order 1] : [scl==1&sda==0] {bit_idx(:) = 8;
      |                 data(:) = 0;}
  sendAck -> waitEndOfAck : [scl==1]
  getcfgdata -> getcfgregstart [order 1] : [bit_idx > 0]
  getcfgregstart -> getcfgdata : [scl == 1]
  getcfgdata -> sendAck [order 2]
  data: reg function_input; regdata function_output; sda input boolean; scl input boolean; sda_out output boolean; addr local fixdt(0,7,0) size=1; bit_idx local uint8; deviceAddr parameter fixdt(0,7,0); data local fixdt(0,8,0) size=1; rw local boolean; reg_idx local uint8; rd_cnt local uint8; powerRegAddr parameter uint8; AccelXRegAddr parameter uint8; AccelYRegAddr parameter uint8; AccelZRegAddr parameter uint8

== matlab function gm_mpu6050/MATLAB Function ==
  data: in input; addr output
function addr = fcn(in)
    addr = uint8(in);
